simulink library "emily"  (R2017a)
settings: Solver=VariableStepAuto  StartTime=0.0  StopTime=10.0  RelTol=1e-3
values from neighbouring files (symbols this model uses):
  param =     [param.mat]
undefined symbols (not defined in the file or in its folder): annparam, update_wrap
libraries: simulink x3
settings Model: Creator=mitchallain  LastModifiedBy=mitchallain

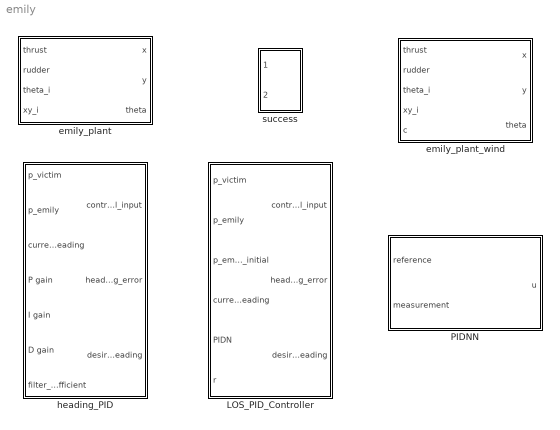
== system emily ==
  LOS_PID_Controller : Subsystem
      settings: AttributesFormatString=%<LinkStatus>
  PIDNN : Subsystem
  emily_plant : Subsystem
  emily_plant_wind : Subsystem
  heading_PID : Subsystem
      settings: AttributesFormatString=%<LinkStatus>
  success : Subsystem

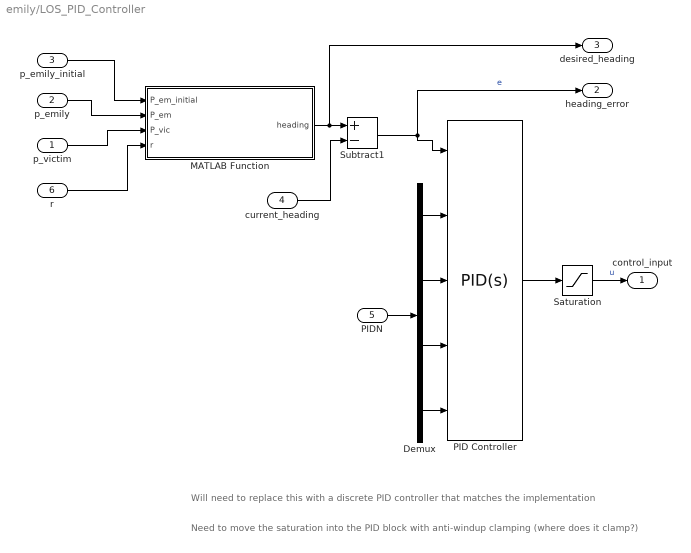
== system emily/LOS_PID_Controller ==
  note: Will need to replace this with a discrete PID controller that matches the implementation
  note: Need to move the saturation into the PID block with anti-windup clamping (where does it clamp?)
  p_victim : Inport
  p_emily : Inport  Port=2
  p_emily_initial : Inport  Port=3
  current_heading : Inport  Port=4
  PIDN : Inport  Port=5
  r : Inport  Port=6
  Demux : Demux
  MATLAB Function : MATLAB Function  TreatAsAtomicUnit=on
  PID Controller : simulink/Continuous/PID Controller  Controller=PID  TimeDomain=Continuous-time  SampleTime=-1  IntegratorMethod=Forward Euler  FilterMethod=Forward Euler  Form=Parallel  UseFilter=on  ControllerParametersSource=external  P=0.01  I=0.0001  D=1  N=100  InitialConditionSource=internal  InitialConditionForIntegrator=0  InitialConditionForFilter=0  ExternalReset=none  LimitOutput=off  UpperSaturationLimit=pi/4  LowerSaturationLimit=-pi/4  LinearizeAsGain=on  AntiWindupMode=clamping  Kb=1  TrackingMode=off  Kt=1  PParamMin=[]  PParamMax=[]  IParamMin=[]  IParamMax=[]  DParamMin=[]  DParamMax=[]  NParamMin=[]  NParamMax=[]  KbParamMin=[]  KbParamMax=[]  KtParamMin=[]  KtParamMax=[]  POutMin=[]  POutMax=[]  IOutMin=[]  IOutMax=[]  DOutMin=[]  DOutMax=[]  NOutMin=[]  NOutMax=[]  KbOutMin=[]  KbOutMax=[]  KtOutMin=[]  KtOutMax=[]  IntegratorOutMin=[]  IntegratorOutMax=[]  FilterOutMin=[]  FilterOutMax=[]  SumOutMin=[]  SumOutMax=[]  SumI1OutMin=[]  SumI1OutMax=[]  SumI2OutMin=[]  SumI2OutMax=[]  SumI3OutMin=[]  SumI3OutMax=[]  SumDOutMin=[]  SumDOutMax=[]  SaturationOutMin=[]  SaturationOutMax=[]  IntegratorContinuousStateAttributes=''  IntegratorStateMustResolveToSignalObject=off  IntegratorRTWStateStorageClass=Auto  FilterContinuousStateAttributes=''  FilterStateMustResolveToSignalObject=off  FilterRTWStateStorageClass=Auto  DifferentiatorICPrevScaledInput=0  DifferentiatorOutMin=[]  DifferentiatorOutMax=[]  InitialConditionSetting=State (most efficient)
  Saturation : Saturate  UpperLimit=pi/4  LowerLimit=-pi/4
  Subtract1 : Sum  Inputs=+-
  control_input : Outport
  heading_error : Outport  Port=2
  desired_heading : Outport  Port=3
  wires:
  Saturation/1 -> control_input/1  "u"
  PID Controller/1 -> Saturation/1
  Subtract1/1 -> heading_error/1, PID Controller/1  "e"
  current_heading/1 -> Subtract1/2
  PIDN/1 -> Demux/1
  Demux/1 -> PID Controller/2
  Demux/2 -> PID Controller/3
  Demux/3 -> PID Controller/4
  Demux/4 -> PID Controller/5
  p_victim/1 -> MATLAB Function/3(P_vic)
  p_emily/1 -> MATLAB Function/2(P_em)
  p_emily_initial/1 -> MATLAB Function/1(P_em_initial)
  r/1 -> MATLAB Function/4(r)
  MATLAB Function/1(heading) -> desired_heading/1, Subtract1/1

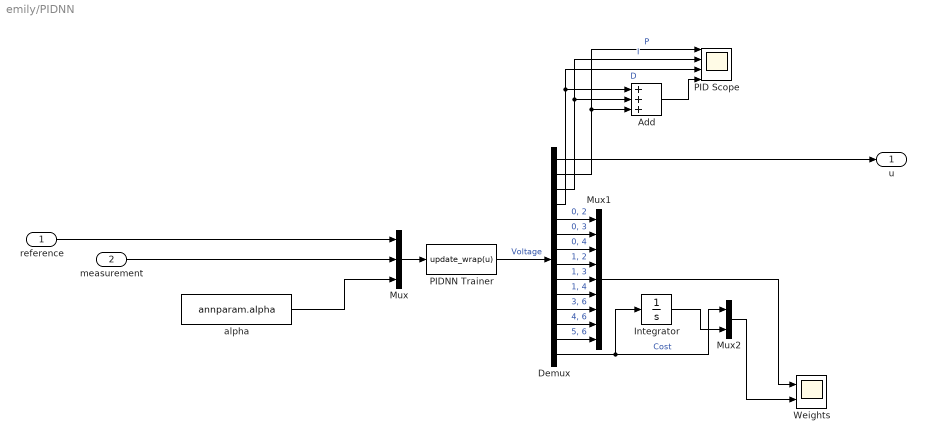
== system emily/PIDNN ==
  reference : Inport
  measurement : Inport  Port=2
  Add : Sum  Inputs=+++
  Demux : Demux  Outputs=14
  Integrator : Integrator
  Mux : Mux  Inputs=3
  Mux1 : Mux  Inputs=9
  Mux2 : Mux  Inputs=2
  PID Scope : Scope  NumInputPorts=4
  PIDNN Trainer : MATLABFcn  MATLABFcn=update_wrap(u)  Output1D=off
  Weights : Scope  NumInputPorts=2
  alpha : Constant  Value=annparam.alpha
  u : Outport
  wires:
  Demux/14 -> Integrator/1, Mux2/1  "Cost"
  Demux/2 -> PID Scope/1, Add/3  "P"
  Demux/9 -> Mux1/5  "1, 3"
  Demux/5 -> Mux1/1  "0, 2"
  PIDNN Trainer/1 -> Demux/1  "Voltage"
  Demux/1 -> u/1
  reference/1 -> Mux/1
  Mux/1 -> PIDNN Trainer/1
  Demux/3 -> PID Scope/2, Add/2  "I"
  Demux/4 -> Add/1, PID Scope/3  "D"
  measurement/1 -> Mux/2
  Demux/8 -> Mux1/4  "1, 2"
  Demux/13 -> Mux1/9  "5, 6"
  Demux/6 -> Mux1/2  "0, 3"
  Demux/12 -> Mux1/8  "4, 6"
  Demux/7 -> Mux1/3  "0, 4"
  Demux/10 -> Mux1/6  "1, 4"
  Mux1/1 -> Weights/1
  Demux/11 -> Mux1/7  "3, 6"
  alpha/1 -> Mux/3
  Add/1 -> PID Scope/4
  Integrator/1 -> Mux2/2
  Mux2/1 -> Weights/2

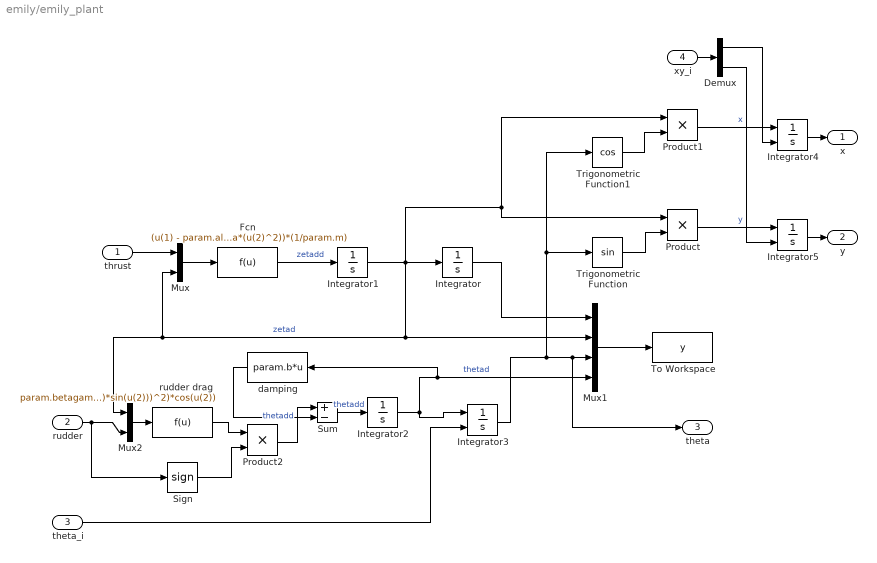
== system emily/emily_plant ==
  thrust : Inport
  rudder : Inport  Port=2
  theta_i : Inport  Port=3
  xy_i : Inport  Port=4
  Demux : Demux  Outputs=2
  Fcn : Fcn  Expr=(u(1) - param.alpha*(u(2)^2))*(1/param.m)
  Integrator : Integrator
  Integrator1 : Integrator
  Integrator2 : Integrator
  Integrator3 : Integrator  InitialConditionSource=external  InitialCondition=5*pi/6  WrapState=on
  Integrator4 : Integrator  InitialConditionSource=external
  Integrator5 : Integrator  InitialConditionSource=external
  Mux : Mux  Inputs=2
  Mux1 : Mux
  Mux2 : Mux  Inputs=2
  Product : Product
  Product1 : Product
  Product2 : Product
  Sign : Signum
  Sum : Sum  Inputs=+-
  To Workspace : ToWorkspace  VariableName=y  SampleTime=-1
  Trigonometric Function : Trigonometry
  Trigonometric Function1 : Trigonometry  Operator=cos
  damping : Fcn  Expr=param.b*u
  rudder drag : Fcn  Expr=param.betagamma*((u(1)*sin(u(2)))^2)*cos(u(2))
  x : Outport
  y : Outport  Port=2
  theta : Outport  Port=3
  wires:
  Mux1/1 -> To Workspace/1
  Integrator/1 -> Mux1/1
  Mux2/1 -> rudder drag/1
  rudder/1 -> Mux2/2, Sign/1
  Sum/1 -> Integrator2/1  "thetadd"
  Integrator2/1 -> Integrator3/1, damping/1, Mux1/4  "thetad"
  Integrator3/1 -> theta/1, Mux1/3, Trigonometric Function1/1, Trigonometric Function/1
  Trigonometric Function/1 -> Product/2
  Trigonometric Function1/1 -> Product1/2
  Product/1 -> Integrator5/1  "y"
  Integrator5/1 -> y/1
  Product1/1 -> Integrator4/1  "x"
  Integrator4/1 -> x/1
  Fcn/1 -> Integrator1/1  "zetadd"
  Mux/1 -> Fcn/1
  thrust/1 -> Mux/1
  Integrator1/1 -> Product1/1, Product/1, Mux2/1, Mux/2, Mux1/2, Integrator/1  "zetad"
  rudder drag/1 -> Product2/1
  Sign/1 -> Product2/2
  theta_i/1 -> Integrator3/2
  Product2/1 -> Sum/1  "thetadd"
  damping/1 -> Sum/2
  xy_i/1 -> Demux/1
  Demux/2 -> Integrator5/2
  Demux/1 -> Integrator4/2

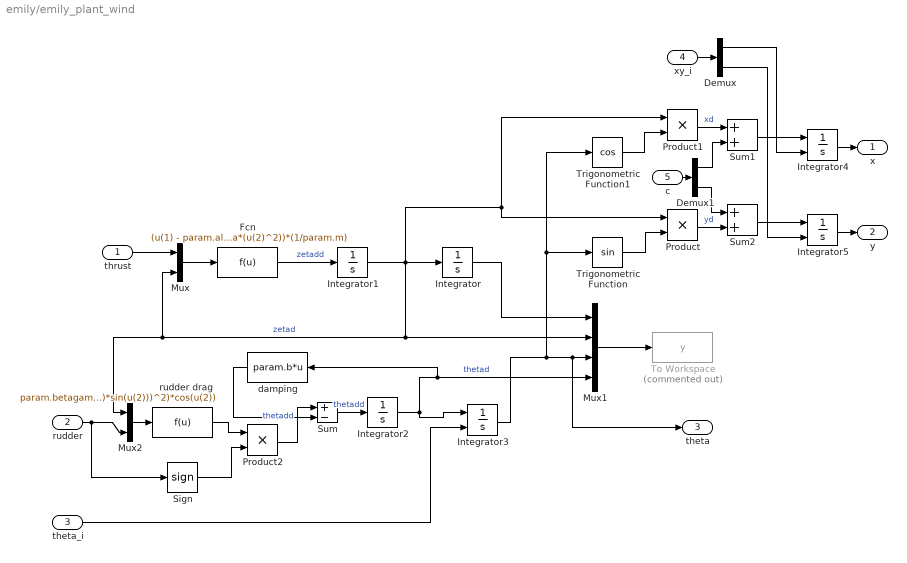
== system emily/emily_plant_wind ==
  thrust : Inport
  rudder : Inport  Port=2
  theta_i : Inport  Port=3
  xy_i : Inport  Port=4
  c : Inport  Port=5
  Demux : Demux  Outputs=2
  Demux1 : Demux  Outputs=2
  Fcn : Fcn  Expr=(u(1) - param.alpha*(u(2)^2))*(1/param.m)
  Integrator : Integrator
  Integrator1 : Integrator
  Integrator2 : Integrator
  Integrator3 : Integrator  InitialConditionSource=external  InitialCondition=5*pi/6  WrapState=on
  Integrator4 : Integrator  InitialConditionSource=external
  Integrator5 : Integrator  InitialConditionSource=external
  Mux : Mux  Inputs=2
  Mux1 : Mux
  Mux2 : Mux  Inputs=2
  Product : Product
  Product1 : Product
  Product2 : Product
  Sign : Signum
  Sum : Sum  Inputs=+-
  Sum1 : Sum
  Sum2 : Sum
  To Workspace : ToWorkspace  Commented=on  VariableName=y  SampleTime=-1
  Trigonometric Function : Trigonometry
  Trigonometric Function1 : Trigonometry  Operator=cos
  damping : Fcn  Expr=param.b*u
  rudder drag : Fcn  Expr=param.betagamma*((u(1)*sin(u(2)))^2)*cos(u(2))
  x : Outport
  y : Outport  Port=2
  theta : Outport  Port=3
  wires:
  Demux/1 -> Integrator4/2
  Demux/2 -> Integrator5/2
  xy_i/1 -> Demux/1
  damping/1 -> Sum/2
  Product2/1 -> Sum/1  "thetadd"
  theta_i/1 -> Integrator3/2
  Sign/1 -> Product2/2
  rudder drag/1 -> Product2/1
  Integrator1/1 -> Integrator/1, Mux1/2, Mux/2, Mux2/1, Product/1, Product1/1  "zetad"
  thrust/1 -> Mux/1
  Mux/1 -> Fcn/1
  Fcn/1 -> Integrator1/1  "zetadd"
  Integrator4/1 -> x/1
  Product1/1 -> Sum1/1  "xd"
  Integrator5/1 -> y/1
  Product/1 -> Sum2/2  "yd"
  Trigonometric Function1/1 -> Product1/2
  Trigonometric Function/1 -> Product/2
  Integrator3/1 -> Trigonometric Function/1, Trigonometric Function1/1, Mux1/3, theta/1
  Integrator2/1 -> Mux1/4, damping/1, Integrator3/1  "thetad"
  Sum/1 -> Integrator2/1  "thetadd"
  rudder/1 -> Sign/1, Mux2/2
  Mux2/1 -> rudder drag/1
  Integrator/1 -> Mux1/1
  Mux1/1 -> To Workspace/1
  c/1 -> Demux1/1
  Demux1/1 -> Sum1/2
  Demux1/2 -> Sum2/1
  Sum2/1 -> Integrator5/1
  Sum1/1 -> Integrator4/1

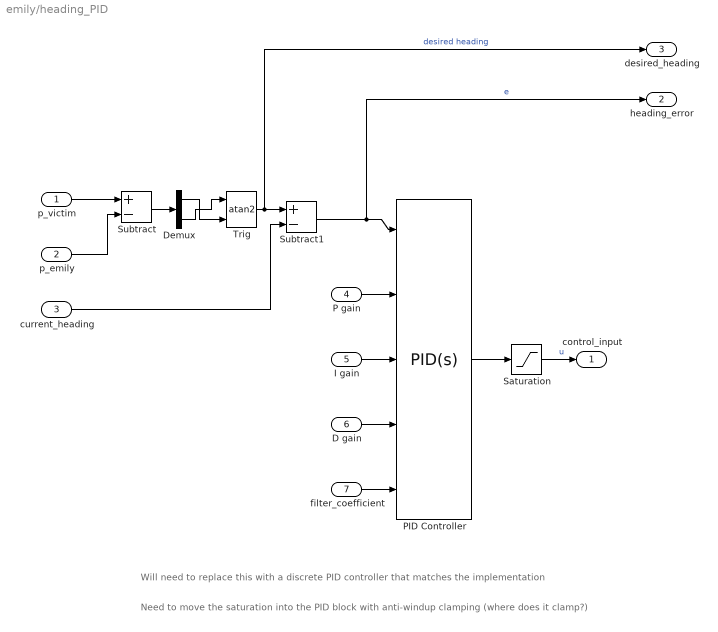
== system emily/heading_PID ==
  note: Will need to replace this with a discrete PID controller that matches the implementation
  note: Need to move the saturation into the PID block with anti-windup clamping (where does it clamp?)
  p_victim : Inport
  p_emily : Inport  Port=2
  current_heading : Inport  Port=3
  P gain : Inport  Port=4
  I gain : Inport  Port=5
  D gain : Inport  Port=6
  filter_coefficient : Inport  Port=7
  Demux : Demux  Outputs=2
  PID Controller : simulink/Continuous/PID Controller  Controller=PID  TimeDomain=Continuous-time  SampleTime=-1  IntegratorMethod=Forward Euler  FilterMethod=Forward Euler  Form=Parallel  UseFilter=on  ControllerParametersSource=external  P=0.01  I=0.0001  D=1  N=100  InitialConditionSource=internal  InitialConditionForIntegrator=0  InitialConditionForFilter=0  ExternalReset=none  LimitOutput=off  UpperSaturationLimit=pi/4  LowerSaturationLimit=-pi/4  LinearizeAsGain=on  AntiWindupMode=clamping  Kb=1  TrackingMode=off  Kt=1  PParamMin=[]  PParamMax=[]  IParamMin=[]  IParamMax=[]  DParamMin=[]  DParamMax=[]  NParamMin=[]  NParamMax=[]  KbParamMin=[]  KbParamMax=[]  KtParamMin=[]  KtParamMax=[]  POutMin=[]  POutMax=[]  IOutMin=[]  IOutMax=[]  DOutMin=[]  DOutMax=[]  NOutMin=[]  NOutMax=[]  KbOutMin=[]  KbOutMax=[]  KtOutMin=[]  KtOutMax=[]  IntegratorOutMin=[]  IntegratorOutMax=[]  FilterOutMin=[]  FilterOutMax=[]  SumOutMin=[]  SumOutMax=[]  SumI1OutMin=[]  SumI1OutMax=[]  SumI2OutMin=[]  SumI2OutMax=[]  SumI3OutMin=[]  SumI3OutMax=[]  SumDOutMin=[]  SumDOutMax=[]  SaturationOutMin=[]  SaturationOutMax=[]  IntegratorContinuousStateAttributes=''  IntegratorStateMustResolveToSignalObject=off  IntegratorRTWStateStorageClass=Auto  FilterContinuousStateAttributes=''  FilterStateMustResolveToSignalObject=off  FilterRTWStateStorageClass=Auto  DifferentiatorICPrevScaledInput=0  DifferentiatorOutMin=[]  DifferentiatorOutMax=[]  InitialConditionSetting=State (most efficient)
  Saturation : Saturate  UpperLimit=pi/4  LowerLimit=-pi/4
  Subtract : Sum  Inputs=+-
  Subtract1 : Sum  Inputs=+-
  "Trig " : Trigonometry  Operator=atan2
  control_input : Outport
  heading_error : Outport  Port=2
  desired_heading : Outport  Port=3
  wires:
  Demux/1 -> "Trig "/2
  Saturation/1 -> control_input/1  "u"
  "Trig "/1 -> desired_heading/1, Subtract1/1  "desired heading"
  p_victim/1 -> Subtract/1
  Subtract/1 -> Demux/1
  p_emily/1 -> Subtract/2
  PID Controller/1 -> Saturation/1
  Demux/2 -> "Trig "/1
  Subtract1/1 -> heading_error/1, PID Controller/1  "e"
  current_heading/1 -> Subtract1/2
  P gain/1 -> PID Controller/2
  I gain/1 -> PID Controller/3
  D gain/1 -> PID Controller/4
  filter_coefficient/1 -> PID Controller/5

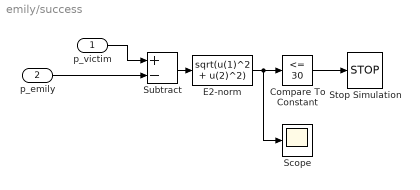
== system emily/success ==
  p_victim : Inport
  p_emily : Inport  Port=2
  Compare To Constant : simulink/Logic and Bit Operations/Compare To Constant  relop=<=  const=30  OutDataTypeStr=boolean
  E2-norm : Fcn  Expr=sqrt(u(1)^2 + u(2)^2)
  Scope : Scope
  Stop Simulation : Stop
  Subtract : Sum  Inputs=+-
  wires:
  p_emily/1 -> Subtract/2
  Compare To Constant/1 -> Stop Simulation/1
  p_victim/1 -> Subtract/1
  E2-norm/1 -> Scope/1, Compare To Constant/1
  Subtract/1 -> E2-norm/1

== matlab function emily/LOS_PID_Controller/MATLAB Function ==
  data: P_em_initial input; heading output; P_em input; P_vic input; r input
function heading  = straightpathLOS(P_em_initial, P_em, P_vic, r)
% This function computes the heading angle according to LOS geometric law
%   Assumes straight line path from initial location to victim
%   If two intersections are produced, the intersection with a higher
%   dispacement parameter (s) is chosen (i.e., farther along path)

% Args:
%   P_em_initial (2-vector): initial (x, y) location of EMILY
%   P_em (2-vector): current (x, y) location of EMILY
%   P_vic (2-vector): victim (x, y) location
%   r (float): radius for LOS control

% Returns:
%   heading: heading angle for EMILY in global frame

% Compute vector from initial EMILY to victim in global frame
P_eiv = P_vic - P_em_initial;

% Compute desired path length and angle
d = norm(P_eiv);
path_angle = atan2(P_eiv(2), P_eiv(1));

% Compute vector from current EMILY to victim
P_ev = P_vic - P_em;

% Bearing is used to seed the fminsearch
bearing = atan2(P_ev(2), P_ev(1));

% Parameterized straight path
xpath = @(s) P_em_initial(1) + s*cos(path_angle);
ypath = @(s) P_em_initial(2) + s*sin(path_angle);

% Parameterized circle about emily
xLOS = @(phi) P_em(1) + r*cos(phi);
yLOS = @(phi) P_em(2) + r*sin(phi);

% Sum of square difference on both axes
xy = @(param) (xpath(param(1)) - xLOS(param(2)))^2 + (ypath(param(1)) - yLOS(param(2)))^2;

% Run fminsearch with IC's as full distance of path and bearing directly to
% victim
temp = fminsearch(@(param) xy(param), [d, bearing]);
s_i = temp(1);
phi_i = temp(2);

% Vector from emily to intersection, P_es
P_es = [xpath(s_i) - P_em(1); ypath(s_i) - P_em(2)];
heading = atan2(P_es(2), P_es(1));

end
